simulink model "model"  (R2020a)
settings: Solver=FixedStepDiscrete  StartTime=0.0  StopTime=10e-6  FixedStep=model_params.ts  RelTol=1e-3
undefined symbols (not defined in the file or in its folder): model_params
settings Model: DataTypeOverride=Off  Creator=glavigna  LastModifiedBy=glavigna
settings OptimizationCC: BlockReduction=off  ConditionallyExecuteInputs=off  DefaultParameterBehavior=Inlined
settings DebuggingCC: AlgebraicLoopMsg=error  SingleTaskRateTransMsg=error
settings HardwareCC: ProdBitPerPointer=32  ProdBitPerSizeT=32  ProdBitPerPtrDiffT=32  ProdLargestAtomicFloat=None  ProdIntDivRoundTo=Undefined  ProdEndianess=Unspecified  ProdWordSize=32  ProdHWDeviceType=ASIC/FPGA->ASIC/FPGA  TargetBitPerPointer=64  TargetBitPerSizeT=64  TargetBitPerPtrDiffT=64  TargetLongLongMode=on  TargetIntDivRoundTo=Zero  TargetEndianess=LittleEndian  TargetWordSize=64  TargetHWDeviceType=Custom Processor->MATLAB Host Computer  ProdEqTarget=off

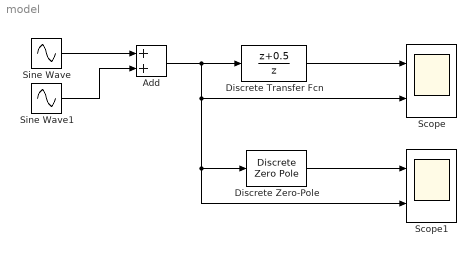
== system model ==
  Add : Sum
  Discrete Transfer Fcn : DiscreteTransferFcn  Numerator=[1 0.5]  Denominator=[1 0]  SampleTime=model_params.ts  a0EqualsOne=on
  Discrete Zero-Pole : DiscreteZeroPole  Zeros=[-0.5]  Poles=[0]  Gain=1  SampleTime=-1
  Scope : Scope  NumInputPorts=2
  Scope1 : Scope  NumInputPorts=2
  Sine Wave : Sin  Frequency=0.2*model_params.fs  SampleTime=model_params.ts
  Sine Wave1 : Sin  Frequency=2*0.9*pi*model_params.fs  SampleTime=model_params.ts
  wires:
  Sine Wave/1 -> Add/1
  Discrete Transfer Fcn/1 -> Scope/1
  Discrete Zero-Pole/1 -> Scope1/1
  Sine Wave1/1 -> Add/2
  Add/1 -> Scope1/2, Discrete Zero-Pole/1, Scope/2, Discrete Transfer Fcn/1
